simulink model "ModelCreation"  (R2023b)
settings: Solver=FixedStepAuto  StartTime=0.0  StopTime=30  RelTol=1e-3
InitFcn:
  | if exist('recordedSignals1', 'var')
  |     disp('recordedSignals1 exists!');
  | else
  |     ModelCreationSignalsLoader; % tune PID using systune
  | end
libraries: Motor x8, simulink x1
settings Model: Creator=Alex  LastModifiedBy=Alex

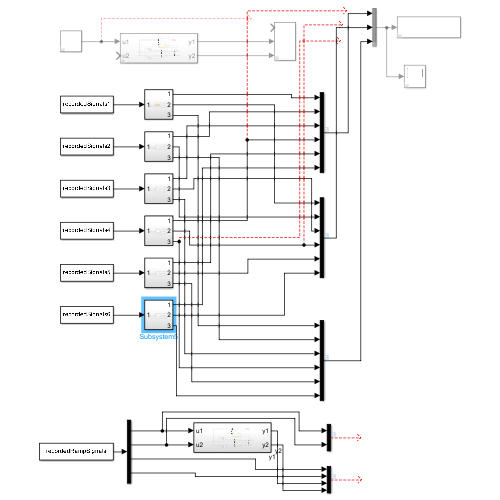
[thumbnail: Simulink's stored preview of the top-level diagram]
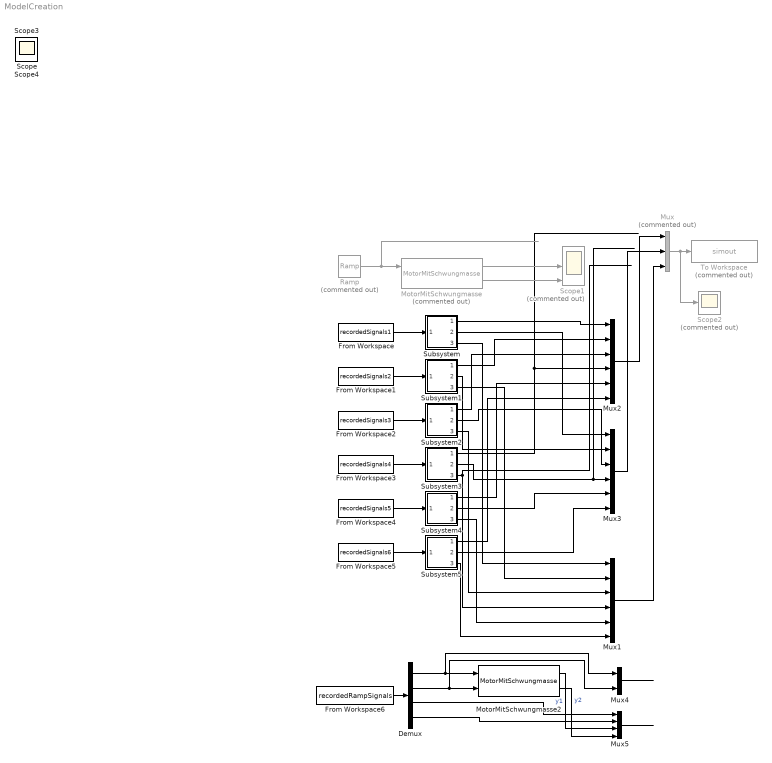
== system ModelCreation ==
  Demux : Demux
  From Workspace : FromWorkspace  VariableName=recordedSignals1  SampleTime=0.01
  From Workspace1 : FromWorkspace  VariableName=recordedSignals2
  From Workspace2 : FromWorkspace  VariableName=recordedSignals3
  From Workspace3 : FromWorkspace  VariableName=recordedSignals4
  From Workspace4 : FromWorkspace  VariableName=recordedSignals5
  From Workspace5 : FromWorkspace  VariableName=recordedSignals6
  From Workspace6 : FromWorkspace  VariableName=recordedRampSignals  SampleTime=0.01
  MotorMitSchwungmasse : Motor/MotorMitSchwungmasse  Commented=on  SystemSampleTime=-1  VariantActivationTime=update diagram  AllowFlexibleInterface=on  Latency=0  AutoFrameSizeCalculation=off
  MotorMitSchwungmasse2 : Motor/MotorMitSchwungmasse  SystemSampleTime=-1  VariantActivationTime=update diagram  AllowFlexibleInterface=on  Latency=0  AutoFrameSizeCalculation=off
  Mux : Mux  Commented=on  Inputs=3
  Mux1 : Mux  Inputs=6
  Mux2 : Mux  Inputs=6
  Mux3 : Mux  Inputs=6
  Mux4 : Mux  Inputs=2
  Mux5 : Mux
  Ramp : simulink/Sources/Ramp  Commented=on  slope=100  start=0  InitialOutput=0
  Scope1 : Scope  Commented=on  NumInputPorts=3
  Scope2 : Scope  Commented=on
  Subsystem : Subsystem
  Subsystem1 : Subsystem
  Subsystem2 : Subsystem
  Subsystem3 : Subsystem
  Subsystem4 : Subsystem
  Subsystem5 : Subsystem
  To Workspace : ToWorkspace  Commented=on  VariableName=simout  SaveFormat=Timeseries  SampleTime=-1
  Scope : Scope
  Scope3 : Scope
  Scope4 : Scope
  wires:
  Subsystem/1(Out1) -> Mux2/1
  Mux2/1 -> Mux/1
  From Workspace1/1 -> Subsystem1/1(In1)
  Subsystem1/1(Out1) -> Mux2/2
  From Workspace/1 -> Subsystem/1(In1)
  Subsystem/2(Out2) -> Mux3/1
  Subsystem1/2(Out2) -> Mux3/2
  From Workspace2/1 -> Subsystem2/1(In1)
  From Workspace3/1 -> Subsystem3/1(In1)
  From Workspace4/1 -> Subsystem4/1(In1)
  From Workspace5/1 -> Subsystem5/1(In1)
  Subsystem2/1(Out1) -> Mux2/3
  Subsystem2/2(Out2) -> Mux3/3
  Subsystem3/1(Out1) -> Mux2/4
  Subsystem3/2(Out2) -> Mux3/4
  Subsystem4/1(Out1) -> Mux2/5
  Subsystem4/2(Out2) -> Mux3/5
  Subsystem5/1(Out1) -> Mux2/6
  Subsystem5/2(Out2) -> Mux3/6
  Mux3/1 -> Mux/2
  Subsystem/3(Out3) -> Mux1/1
  Subsystem1/3(Out3) -> Mux1/2
  Subsystem2/3(Out3) -> Mux1/3
  Subsystem3/3(Out3) -> Mux1/4
  Subsystem4/3(Out3) -> Mux1/5
  Subsystem5/3(Out3) -> Mux1/6
  Mux1/1 -> Mux/3
  Ramp/1 -> MotorMitSchwungmasse/1
  MotorMitSchwungmasse/2 -> Scope1/3
  MotorMitSchwungmasse/1 -> Scope1/2
  Mux/1 -> Scope2/1, To Workspace/1
  From Workspace6/1 -> Demux/1
  Mux4/1 -> ?
  Mux5/1 -> ?
  Demux/1 -> MotorMitSchwungmasse2/1, Mux4/1
  Demux/2 -> MotorMitSchwungmasse2/2, Mux4/2
  Demux/3 -> Mux5/1
  Demux/4 -> Mux5/2
  MotorMitSchwungmasse2/2 -> Mux5/4  "y2"
  MotorMitSchwungmasse2/1 -> Mux5/3  "y1"

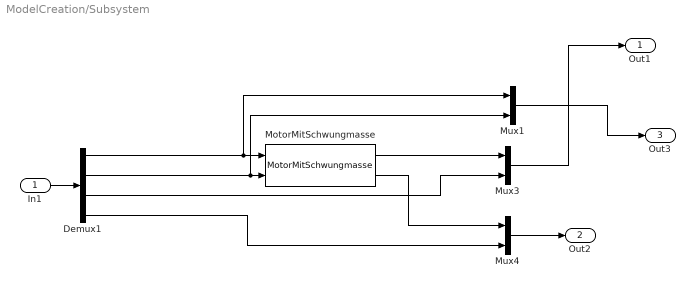
== system ModelCreation/Subsystem ==
  In1 : Inport
  Demux1 : Demux
  MotorMitSchwungmasse : Motor/MotorMitSchwungmasse  SystemSampleTime=-1  VariantActivationTime=update diagram  AllowFlexibleInterface=on  Latency=0  AutoFrameSizeCalculation=off
  Mux1 : Mux  Inputs=2
  Mux3 : Mux  Inputs=2
  Mux4 : Mux  Inputs=2
  Out1 : Outport
  Out2 : Outport  Port=2
  Out3 : Outport  Port=3
  wires:
  Demux1/3 -> Mux3/2
  Demux1/2 -> Mux1/2, MotorMitSchwungmasse/2
  Demux1/1 -> Mux1/1, MotorMitSchwungmasse/1
  In1/1 -> Demux1/1
  MotorMitSchwungmasse/2 -> Mux4/1
  Mux4/1 -> Out2/1
  Demux1/4 -> Mux4/2
  MotorMitSchwungmasse/1 -> Mux3/1
  Mux3/1 -> Out1/1
  Mux1/1 -> Out3/1

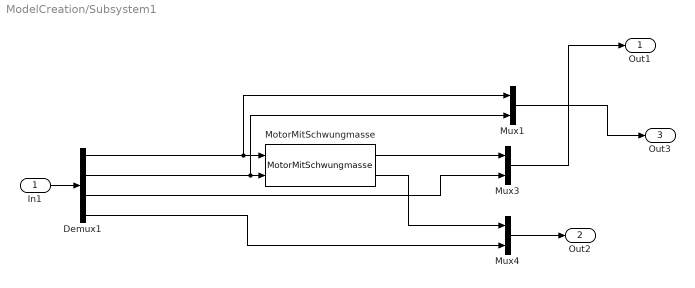
== system ModelCreation/Subsystem1 ==
  In1 : Inport
  Demux1 : Demux
  MotorMitSchwungmasse : Motor/MotorMitSchwungmasse  SystemSampleTime=-1  VariantActivationTime=update diagram  AllowFlexibleInterface=on  Latency=0  AutoFrameSizeCalculation=off
  Mux1 : Mux  Inputs=2
  Mux3 : Mux  Inputs=2
  Mux4 : Mux  Inputs=2
  Out1 : Outport
  Out2 : Outport  Port=2
  Out3 : Outport  Port=3
  wires:
  Demux1/3 -> Mux3/2
  Demux1/2 -> Mux1/2, MotorMitSchwungmasse/2
  Demux1/1 -> Mux1/1, MotorMitSchwungmasse/1
  In1/1 -> Demux1/1
  MotorMitSchwungmasse/2 -> Mux4/1
  Mux4/1 -> Out2/1
  Demux1/4 -> Mux4/2
  MotorMitSchwungmasse/1 -> Mux3/1
  Mux3/1 -> Out1/1
  Mux1/1 -> Out3/1

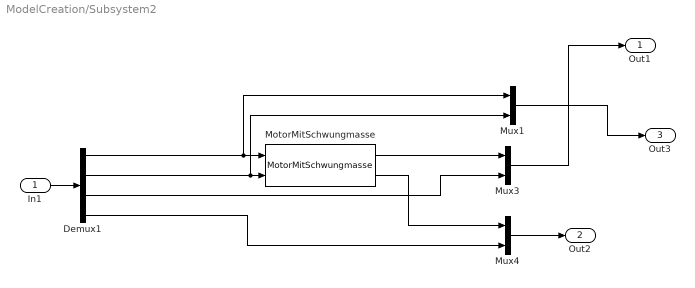
== system ModelCreation/Subsystem2 ==
  In1 : Inport
  Demux1 : Demux
  MotorMitSchwungmasse : Motor/MotorMitSchwungmasse  SystemSampleTime=-1  VariantActivationTime=update diagram  AllowFlexibleInterface=on  Latency=0  AutoFrameSizeCalculation=off
  Mux1 : Mux  Inputs=2
  Mux3 : Mux  Inputs=2
  Mux4 : Mux  Inputs=2
  Out1 : Outport
  Out2 : Outport  Port=2
  Out3 : Outport  Port=3
  wires:
  Demux1/3 -> Mux3/2
  Demux1/2 -> Mux1/2, MotorMitSchwungmasse/2
  Demux1/1 -> Mux1/1, MotorMitSchwungmasse/1
  In1/1 -> Demux1/1
  MotorMitSchwungmasse/2 -> Mux4/1
  Mux4/1 -> Out2/1
  Demux1/4 -> Mux4/2
  MotorMitSchwungmasse/1 -> Mux3/1
  Mux3/1 -> Out1/1
  Mux1/1 -> Out3/1

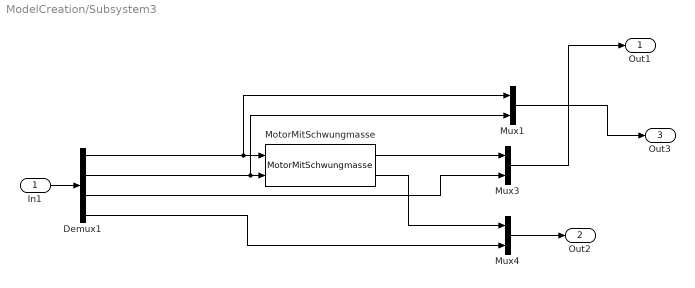
== system ModelCreation/Subsystem3 ==
  In1 : Inport
  Demux1 : Demux
  MotorMitSchwungmasse : Motor/MotorMitSchwungmasse  SystemSampleTime=-1  VariantActivationTime=update diagram  AllowFlexibleInterface=on  Latency=0  AutoFrameSizeCalculation=off
  Mux1 : Mux  Inputs=2
  Mux3 : Mux  Inputs=2
  Mux4 : Mux  Inputs=2
  Out1 : Outport
  Out2 : Outport  Port=2
  Out3 : Outport  Port=3
  wires:
  Demux1/3 -> Mux3/2
  Demux1/2 -> Mux1/2, MotorMitSchwungmasse/2
  Demux1/1 -> Mux1/1, MotorMitSchwungmasse/1
  In1/1 -> Demux1/1
  MotorMitSchwungmasse/2 -> Mux4/1
  Mux4/1 -> Out2/1
  Demux1/4 -> Mux4/2
  MotorMitSchwungmasse/1 -> Mux3/1
  Mux3/1 -> Out1/1
  Mux1/1 -> Out3/1

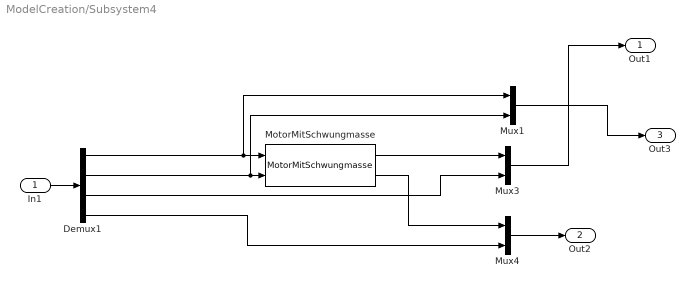
== system ModelCreation/Subsystem4 ==
  In1 : Inport
  Demux1 : Demux
  MotorMitSchwungmasse : Motor/MotorMitSchwungmasse  SystemSampleTime=-1  VariantActivationTime=update diagram  AllowFlexibleInterface=on  Latency=0  AutoFrameSizeCalculation=off
  Mux1 : Mux  Inputs=2
  Mux3 : Mux  Inputs=2
  Mux4 : Mux  Inputs=2
  Out1 : Outport
  Out2 : Outport  Port=2
  Out3 : Outport  Port=3
  wires:
  Demux1/3 -> Mux3/2
  Demux1/2 -> Mux1/2, MotorMitSchwungmasse/2
  Demux1/1 -> Mux1/1, MotorMitSchwungmasse/1
  In1/1 -> Demux1/1
  MotorMitSchwungmasse/2 -> Mux4/1
  Mux4/1 -> Out2/1
  Demux1/4 -> Mux4/2
  MotorMitSchwungmasse/1 -> Mux3/1
  Mux3/1 -> Out1/1
  Mux1/1 -> Out3/1

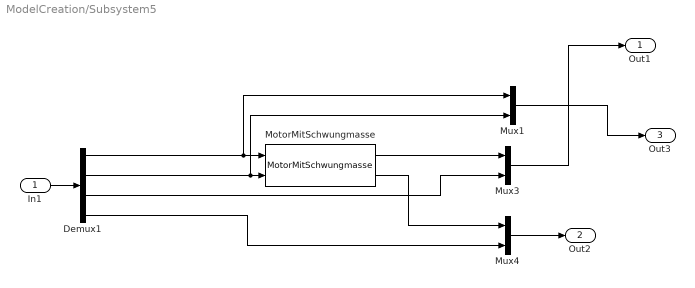
== system ModelCreation/Subsystem5 ==
  In1 : Inport
  Demux1 : Demux
  MotorMitSchwungmasse : Motor/MotorMitSchwungmasse  SystemSampleTime=-1  VariantActivationTime=update diagram  AllowFlexibleInterface=on  Latency=0  AutoFrameSizeCalculation=off
  Mux1 : Mux  Inputs=2
  Mux3 : Mux  Inputs=2
  Mux4 : Mux  Inputs=2
  Out1 : Outport
  Out2 : Outport  Port=2
  Out3 : Outport  Port=3
  wires:
  Demux1/3 -> Mux3/2
  Demux1/2 -> Mux1/2, MotorMitSchwungmasse/2
  Demux1/1 -> Mux1/1, MotorMitSchwungmasse/1
  In1/1 -> Demux1/1
  MotorMitSchwungmasse/2 -> Mux4/1
  Mux4/1 -> Out2/1
  Demux1/4 -> Mux4/2
  MotorMitSchwungmasse/1 -> Mux3/1
  Mux3/1 -> Out1/1
  Mux1/1 -> Out3/1
